simulink model "boiler"  (Simulink 7.8)
settings: Solver=ode45  StartTime=0.0  StopTime=20  RelTol=1e-3
libraries: simulink x1
settings Model: Creator=Max  LastModifiedBy=Max

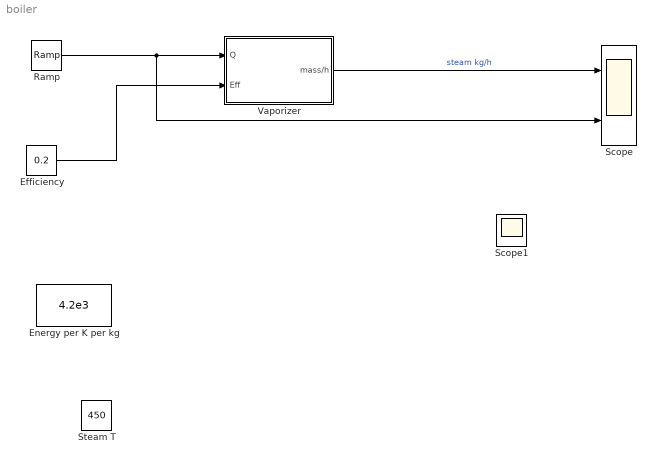
== system boiler ==
  Efficiency : Constant  Value=0.2
  Energy per K per kg : Constant  Value=4.2e3
  Ramp : simulink/Sources/Ramp  slope=5e9  start=0  X0=0
  Scope : Scope  NumInputPorts=2
      settings: TimeRange=20  YMin=0~-5  YMax=25000~5
  Scope1 : Scope
  Steam T : Constant  Value=450
  Vaporizer : Subsystem  TreatAsAtomicUnit=on
  wires:
  Ramp/1 -> Vaporizer/1(Q), Scope/2
  Vaporizer/1(mass/h) -> Scope/1  "steam kg/h"
  Efficiency/1 -> Vaporizer/2(Eff)

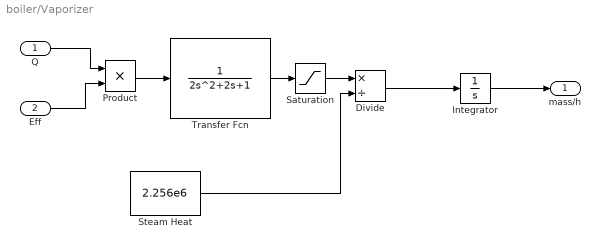
== system boiler/Vaporizer ==
  Q : Inport
  Eff : Inport  Port=2
  Divide : Product  Inputs=*/
  Integrator : Integrator
  Product : Product  RndMeth=Zero
  Saturation : Saturate  UpperLimit=3e9  LowerLimit=0
  Steam Heat : Constant  Value=2.256e6
  Transfer Fcn : TransferFcn  Denominator=[2 2 1]
  mass/h : Outport
  wires:
  Steam Heat/1 -> Divide/2
  Transfer Fcn/1 -> Saturation/1
  Divide/1 -> Integrator/1
  Product/1 -> Transfer Fcn/1
  Q/1 -> Product/1
  Eff/1 -> Product/2
  Integrator/1 -> mass/h/1
  Saturation/1 -> Divide/1
